simulink model "robot_main"  (R2023a)
settings: Solver=VariableStepAuto  StartTime=0.0  StopTime=10.0  RelTol=1e-3
undefined symbols (not defined in the file or in its folder): join_1_pos, join_2_pos, join_3_pos, join_4_pos, join_5_pos, join_6_pos
libraries: sm_lib x2, nesl_utility x1
settings Model: Creator=motya  LastModifiedBy=motya

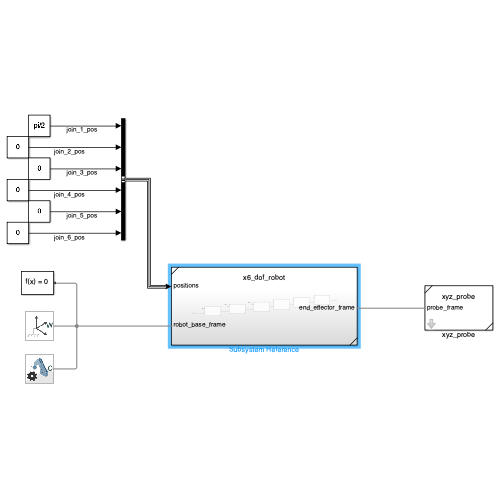
[thumbnail: Simulink's stored preview of the top-level diagram]
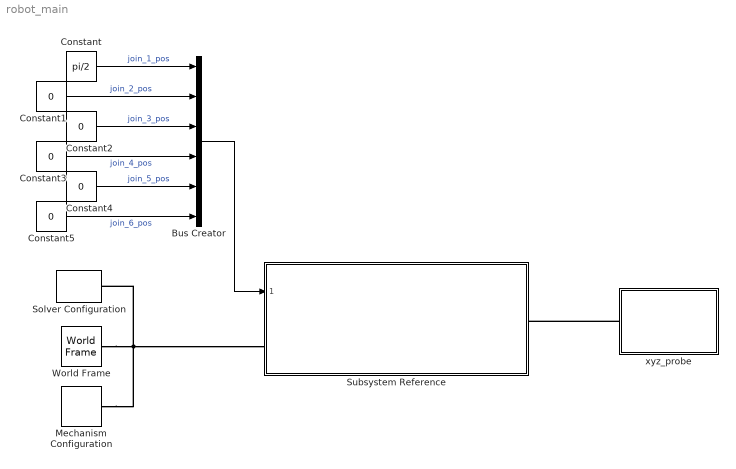
== system robot_main ==
  Bus Creator : BusCreator  Inputs=join_1_pos,join_2_pos,join_3_pos,join_4_pos,join_5_pos,join_6_pos
  Constant : Constant  Value=pi/2
  Constant{1..5} (5 alike) : Constant  Value=0
  Mechanism Configuration : sm_lib/Utilities/Mechanism Configuration  UniformGravity=Constant  GravityVector=[0 0 -9.80665]  GravityVectorUnits=m/s^2  LinearizationDelta=0.001  JointModeTransitionNonlinearIterations=2
  Solver Configuration : nesl_utility/Solver Configuration  PhysicalDomain=network_engine_domain  SubClassName=solver  LeftPortType=input  RightPortType=generic  Tones=[]  Harmonics=[]  SimulateNoise=off  Profile=off  UseLocalSampling=off  EnableSwitchedLinearOptims=on  FrequencyDomain=off  UseCCode=off  RelTol=0.001  AbsTol=0.001  MinStep=1e-09  ToWorkspace=off  RevertToSquareIcSolve=off  NumHomotopyIterations=100  PhasorMode=off  PhasorModeNumHarmonics=1  ConsistencySolver=NEWTON_XTOL_AFTER_FTOL  IndexReductionMethod=DerivativeReplacement  DoDC=off  ResidualTolerance=1e-09  ConsistencyTolSource=GLOBAL  ConsistencyAbsTol=0.001  ConsistencyRelTol=0.001  ConsistencyTolFactor=0.001  UseLocalSolver=off  LocalSolverChoice=NE_TRAPEZOIDAL_ADVANCER  ResolveIndetEquations=on  FunctionEvalNumThread=1  LocalSolverSampleTime=0.001  DoFixedCost=off  MaxNonlinIter=3  MaxModeIter=2  ComputeImpulses=off  ImpulseIterations=2  LinearAlgebra=auto  LinearAlgebraNumThread=0  EquationFormulation=NE_TIME_EF  DelaysMemoryBudget=1024  AutomaticFiltering=on  FilteringTimeConstant=0.001  PartitionStorageMethod=AS_NEEDED  PartitionMemoryBudget=1024  PartitionMethod=ROBUST
  Subsystem Reference : Subsystem  ReferencedSubsystem=x6_dof_robot
  World Frame : sm_lib/Frames and Transforms/World Frame
  xyz_probe : Subsystem  ReferencedSubsystem=xyz_probe  axes_length=0.1  axes_radius=0.005  offset_vector=[0; 0; 0]
  wires:
  Constant/1 -> Bus Creator/1  "join_1_pos"
  Constant2/1 -> Bus Creator/3  "join_3_pos"
  Constant5/1 -> Bus Creator/6  "join_6_pos"
  Constant4/1 -> Bus Creator/5  "join_5_pos"
  Constant3/1 -> Bus Creator/4  "join_4_pos"
  Constant1/1 -> Bus Creator/2  "join_2_pos"
  Bus Creator/1 -> Subsystem Reference/1
  connections:
  World Frame/RConn1 -- Solver Configuration/RConn1 -- Mechanism Configuration/RConn1 -- Subsystem Reference/LConn1
  xyz_probe/LConn1 -- Subsystem Reference/RConn1
